simulink library "pwrsysBasic_202301"  (R2018a)
settings: Solver=VariableStepAuto  StartTime=0.0  StopTime=10.0  RelTol=1e-3
values from neighbouring files (symbols this model uses):
  Iap = 1    [SequenceSeparation_script.m]
  Sn = 1.5    [SequenceSeparation_script.m]
  Ts = 1e-6    (= 1e-06)    [SequenceSeparation_script.m]
undefined symbols (not defined in the file or in its folder): DiscIntNeverNeededParam, fn, Kp, tctrl, Uanp
libraries: pwrsysBasic x15, powerlib_meascontrol x12, pwrsysTransf x8, simulink x3
(part 2 of 2)

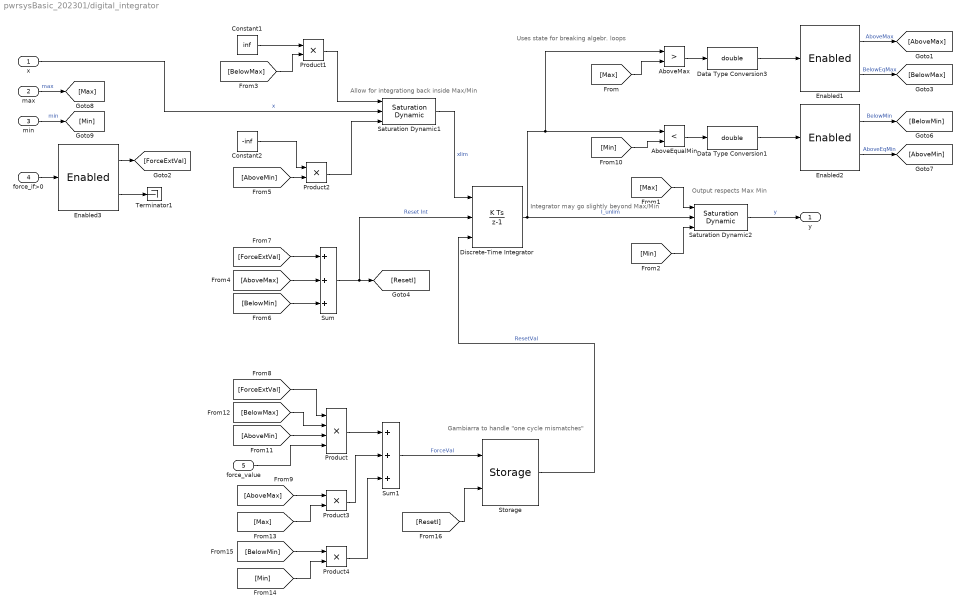
== system pwrsysBasic_202301/digital_integrator ==
  note: Gambiarra to handle "one cycle mismatches"
  note: Integrator may go slightly beyond Max/Min
  note: Output respects Max Min
  note: Uses state for breaking algebr. loops
  note: Allow for integrationg back inside Max/Min
  x : Inport
  max : Inport  Port=2
  min : Inport  Port=3
  force_if>0 : Inport  Port=4
  force_value : Inport  Port=5
  AboveEqualMin : RelationalOperator  Operator=<  OutDataTypeStr=boolean  RndMeth=Nearest
  AboveMax : RelationalOperator  Operator=>  OutDataTypeStr=boolean  RndMeth=Nearest
  Constant1 : Constant  Value=inf
  Constant2 : Constant  Value=-inf
  Data Type Conversion1 : DataTypeConversion  OutDataTypeStr=double
  Data Type Conversion3 : DataTypeConversion  OutDataTypeStr=double
  Discrete-Time Integrator : DiscreteIntegrator  ExternalReset=level  InitialConditionSource=external  SampleTime=Ts  IgnoreLimit=on  ICPrevOutput=DiscIntNeverNeededParam  ICPrevScaledInput=DiscIntNeverNeededParam
  Enabled1 : pwrsysBasic/Enabled
      settings: SourceProductName=NTNU Power Systems
  Enabled2 : pwrsysBasic/Enabled
      settings: SourceProductName=NTNU Power Systems
  Enabled3 : pwrsysBasic/Enabled
      settings: SourceProductName=NTNU Power Systems
  Product : Product  Inputs=4
  Product{1..4} (4 alike) : Product
  Saturation Dynamic1 : simulink/Discontinuities/Saturation Dynamic  OutMin=[]  OutMax=[]  OutDataTypeStr=Inherit: Same as second input  OutDataType=fixdt(1, 16)  OutScaling=2^-10  DoSatur=off
  Saturation Dynamic2 : simulink/Discontinuities/Saturation Dynamic  OutMin=[]  OutMax=[]  OutDataTypeStr=Inherit: Same as second input  OutDataType=fixdt(1, 16)  OutScaling=2^-10  DoSatur=off
  Storage : pwrsysBasic/Storage
      settings: SourceProductName=NTNU Power Systems
  Sum : Sum  Inputs=+++
  Sum1 : Sum  Inputs=+++
  Terminator1 : Terminator
  y : Outport
  wires:
  x/1 -> Saturation Dynamic1/2  "x"
  Saturation Dynamic2/1 -> y/1  "y"
  max/1 -> [Max]  "max"
  min/1 -> [Min]  "min"
  force_value/1 -> Product/4
  Saturation Dynamic1/1 -> Discrete-Time Integrator/1  "xlim"
  [BelowMax] -> Product1/2
  Constant1/1 -> Product1/1
  Product1/1 -> Saturation Dynamic1/1
  [AboveMin] -> Product2/2
  Constant2/1 -> Product2/1
  Product2/1 -> Saturation Dynamic1/3
  Enabled1/1 -> [AboveMax]  "AboveMax"
  Enabled1/2 -> [BelowMax]  "BelowEqMax"
  Enabled2/2 -> [AboveMin]  "AboveEqMin"
  Enabled2/1 -> [BelowMin]  "BelowMin"
  [AboveMax] -> Sum/2
  [BelowMin] -> Sum/3
  force_if>0/1 -> Enabled3/1
  Enabled3/2 -> Terminator1/1
  [ForceExtVal] -> Product/1
  [AboveMax] -> Product3/1
  [Min] -> AboveEqualMin/2
  [AboveMin] -> Product/3
  [BelowMax] -> Product/2
  Product/1 -> Sum1/1
  [Max] -> Product3/2
  [BelowMin] -> Product4/1
  [Min] -> Product4/2
  Product4/1 -> Sum1/3
  Product3/1 -> Sum1/2
  Sum1/1 -> Storage/1  "ForceVal"
  Enabled3/1 -> [ForceExtVal]
  [Max] -> AboveMax/2
  Discrete-Time Integrator/1 -> Saturation Dynamic2/2, AboveEqualMin/1, AboveMax/1  "I_unlim"
  [Max] -> Saturation Dynamic2/1
  [Min] -> Saturation Dynamic2/3
  AboveMax/1 -> Data Type Conversion3/1
  AboveEqualMin/1 -> Data Type Conversion1/1
  Data Type Conversion3/1 -> Enabled1/1
  Data Type Conversion1/1 -> Enabled2/1
  [ForceExtVal] -> Sum/1
  Sum/1 -> Discrete-Time Integrator/2, [ResetI]  "Reset Int"
  [ResetI] -> Storage/2
  Storage/1 -> Discrete-Time Integrator/3  "ResetVal"

== system pwrsysBasic_202301/digital_ramp_gen ==
  up_if>0 : Inport
  down_if>0 : Inport  Port=2
  rate_pu/s : Inport  Port=3
  max : Inport  Port=4
  min : Inport  Port=5
  force_if=1 : Inport  Port=6
  force_value : Inport  Port=7
  Constant : Constant  Value=Ts
  MATLAB Function : MATLAB Function  TreatAsAtomicUnit=on  SystemSampleTime=Ts
      settings: RTWSystemCode=Inline
  y : Outport
  wires:
  up_if>0/1 -> MATLAB Function/1(up)
  MATLAB Function/1(y) -> y/1
  max/1 -> MATLAB Function/4(max)
  min/1 -> MATLAB Function/5(min)
  force_if=1/1 -> MATLAB Function/6(force)
  force_value/1 -> MATLAB Function/7(forceval)
  Constant/1 -> MATLAB Function/8(Ts)
  down_if>0/1 -> MATLAB Function/2(down)
  rate_pu/s/1 -> MATLAB Function/3(rate)

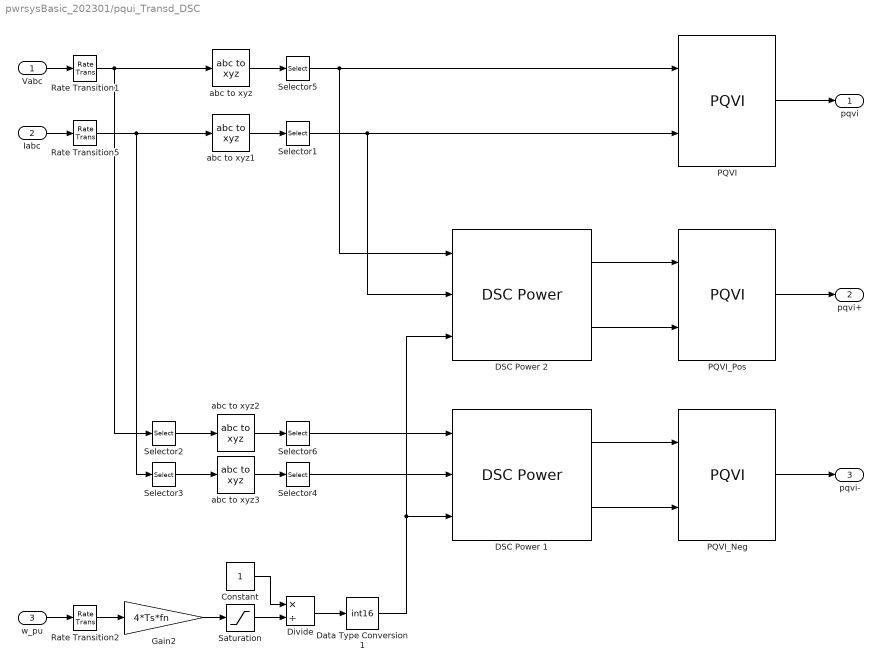
== system pwrsysBasic_202301/pqui_Transd_DSC ==
  Vabc : Inport
  Iabc : Inport  Port=2
  w_pu : Inport  Port=3
  Constant : Constant
  DSC Power 1 : pwrsysBasic/DSC Power 
      settings: SourceProductName=NTNU Power Systems
  DSC Power 2 : pwrsysBasic/DSC Power 
      settings: SourceProductName=NTNU Power Systems
  Data Type Conversion1 : DataTypeConversion  OutDataTypeStr=int16  RndMeth=Round  SaturateOnIntegerOverflow=on
  Divide : Product  Inputs=*/
  Gain2 : Gain  Gain=4*Ts*fn
  PQVI : pwrsysBasic/PQVI  Sn=Sn  Uanp=Uanp  Iap=Iap
      settings: SourceProductName=NTNU Power Systems
  PQVI_Neg : pwrsysBasic/PQVI  Sn=Sn  Uanp=Uanp  Iap=Iap
      settings: SourceProductName=NTNU Power Systems
  PQVI_Pos : pwrsysBasic/PQVI  Sn=Sn  Uanp=Uanp  Iap=Iap
      settings: SourceProductName=NTNU Power Systems
  Rate Transition1 : RateTransition  OutPortSampleTime=Ts
  Rate Transition2 : RateTransition  InitialCondition=1  OutPortSampleTime=Ts
  Rate Transition5 : RateTransition  OutPortSampleTime=Ts
  Saturation : Saturate  UpperLimit=inf  LowerLimit=0.000001
  Selector{1,4..6} (4 alike) : Selector  InputPortWidth=3  IndexOptions=Index vector (dialog)  Indices=[1 2]  OutputSizes=1
  Selector2 : Selector  InputPortWidth=3  IndexOptions=Index vector (dialog)  Indices=[1 3 2]  OutputSizes=1
  Selector3 : Selector  InputPortWidth=3  IndexOptions=Index vector (dialog)  Indices=[1 3 2]  OutputSizes=1
  abc to xyz{,1..3} (4 alike) : pwrsysTransf/abc to xyz  typeTransf=Amplitude-invariant
      settings: SourceProductName=NTNU Power Systems
  pqvi : Outport
  pqvi+ : Outport  Port=2
  pqvi- : Outport  Port=3
  wires:
  abc to xyz1/1 -> Selector1/1
  Vabc/1 -> Rate Transition1/1
  Iabc/1 -> Rate Transition5/1
  Rate Transition1/1 -> abc to xyz/1, Selector2/1
  Rate Transition5/1 -> abc to xyz1/1, Selector3/1
  Selector5/1 -> DSC Power 2/1, PQVI/1
  Selector1/1 -> DSC Power 2/2, PQVI/2
  PQVI/1 -> pqvi/1
  Data Type Conversion1/1 -> DSC Power 1/3, DSC Power 2/3
  DSC Power 2/1 -> PQVI_Pos/1
  DSC Power 2/2 -> PQVI_Pos/2
  PQVI_Pos/1 -> pqvi+/1
  abc to xyz2/1 -> Selector6/1
  abc to xyz3/1 -> Selector4/1
  Selector2/1 -> abc to xyz2/1
  Selector3/1 -> abc to xyz3/1
  Selector6/1 -> DSC Power 1/1
  Selector4/1 -> DSC Power 1/2
  PQVI_Neg/1 -> pqvi-/1
  DSC Power 1/2 -> PQVI_Neg/2
  DSC Power 1/1 -> PQVI_Neg/1
  Saturation/1 -> Divide/2
  Constant/1 -> Divide/1
  Rate Transition2/1 -> Gain2/1
  w_pu/1 -> Rate Transition2/1
  Gain2/1 -> Saturation/1
  Divide/1 -> Data Type Conversion1/1
  abc to xyz/1 -> Selector5/1

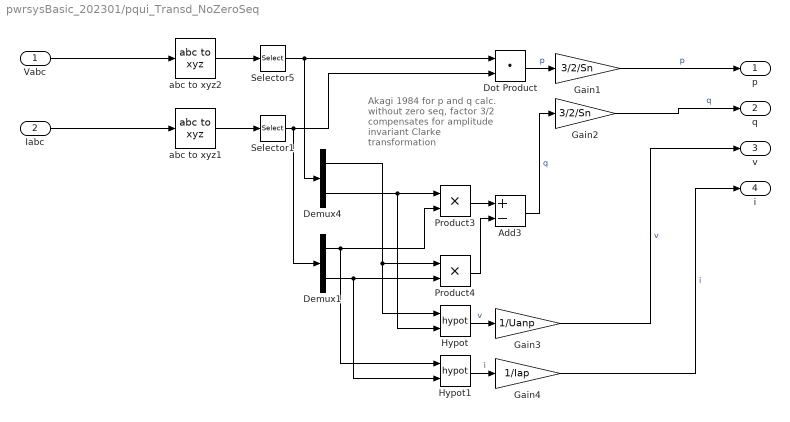
== system pwrsysBasic_202301/pqui_Transd_NoZeroSeq ==
  note: Akagi 1984 for p and q
      | calc. without zero seq,
      | factor 3/2 compensates for
      | amplitude invariant
      | Clarke transformation
  Vabc : Inport
  Iabc : Inport  Port=2
  Add3 : Sum  Inputs=+-
  Demux1 : Demux  Outputs=2
  Demux4 : Demux  Outputs=2
  Dot Product : DotProduct  InputSameDT=on  OutDataTypeStr=Inherit: Inherit via internal rule
  Gain1 : Gain  Gain=3/2/Sn
  Gain2 : Gain  Gain=3/2/Sn
  Gain3 : Gain  Gain=1/Uanp
  Gain4 : Gain  Gain=1/Iap
  Hypot : Math  Operator=hypot  RndMeth=Zero  SaturateOnIntegerOverflow=on
  Hypot1 : Math  Operator=hypot  RndMeth=Zero  SaturateOnIntegerOverflow=on
  Product3 : Product
  Product4 : Product
  Selector1 : Selector  InputPortWidth=3  IndexOptions=Index vector (dialog)  Indices=[1 2]  OutputSizes=1
  Selector5 : Selector  InputPortWidth=3  IndexOptions=Index vector (dialog)  Indices=[1 2]  OutputSizes=1
  abc to xyz1 : pwrsysTransf/abc to xyz  typeTransf=Amplitude-invariant
      settings: SourceProductName=NTNU Power Systems
  abc to xyz2 : pwrsysTransf/abc to xyz  typeTransf=Amplitude-invariant
      settings: SourceProductName=NTNU Power Systems
  p : Outport
  q : Outport  Port=2
  v : Outport  Port=3
  i : Outport  Port=4
  wires:
  abc to xyz1/1 -> Selector1/1
  Gain3/1 -> v/1  "v"
  Demux1/2 -> Hypot1/2, Product4/2
  Hypot1/1 -> Gain4/1  "i"
  Selector1/1 -> Demux1/1, Dot Product/2
  Selector5/1 -> Demux4/1, Dot Product/1
  Demux4/1 -> Hypot/1, Product4/1
  Hypot/1 -> Gain3/1  "v"
  Dot Product/1 -> Gain1/1  "p"
  Demux1/1 -> Hypot1/1, Product3/2
  Add3/1 -> Gain2/1  "q"
  Product4/1 -> Add3/2
  Demux4/2 -> Hypot/2, Product3/1
  Vabc/1 -> abc to xyz2/1
  abc to xyz2/1 -> Selector5/1
  Iabc/1 -> abc to xyz1/1
  Product3/1 -> Add3/1
  Gain1/1 -> p/1  "p"
  Gain4/1 -> i/1  "i"
  Gain2/1 -> q/1  "q"

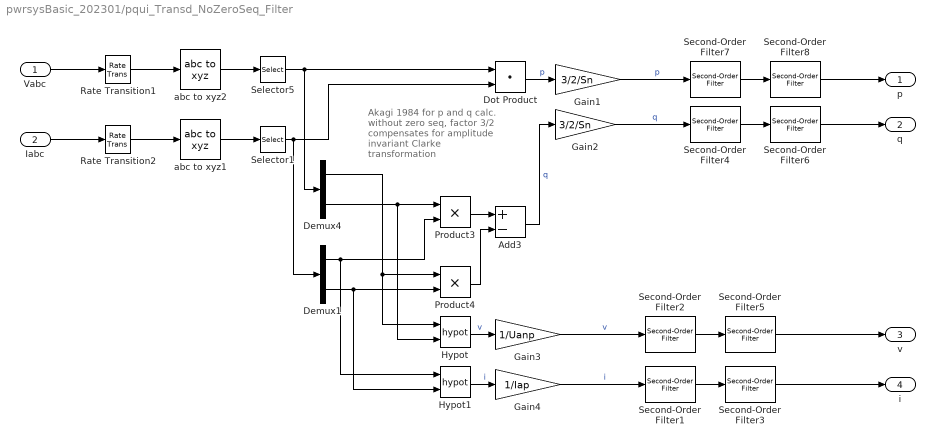
== system pwrsysBasic_202301/pqui_Transd_NoZeroSeq_Filter ==
  note: Akagi 1984 for p and q
      | calc. without zero seq,
      | factor 3/2 compensates for
      | amplitude invariant
      | Clarke transformation
  Vabc : Inport
  Iabc : Inport  Port=2
  Add3 : Sum  Inputs=+-
  Demux1 : Demux  Outputs=2
  Demux4 : Demux  Outputs=2
  Dot Product : DotProduct  InputSameDT=on  OutDataTypeStr=Inherit: Inherit via internal rule
  Gain1 : Gain  Gain=3/2/Sn
  Gain2 : Gain  Gain=3/2/Sn
  Gain3 : Gain  Gain=1/Uanp
  Gain4 : Gain  Gain=1/Iap
  Hypot : Math  Operator=hypot  RndMeth=Zero  SaturateOnIntegerOverflow=on
  Hypot1 : Math  Operator=hypot  RndMeth=Zero  SaturateOnIntegerOverflow=on
  Product3 : Product
  Product4 : Product
  Rate Transition1 : RateTransition  OutPortSampleTime=Ts
  Rate Transition2 : RateTransition  OutPortSampleTime=Ts
  Second-Order Filter1 : powerlib_meascontrol/Filters/Second-Order Filter  FilterType=Lowpass  Fo=fcutoutvi  Zeta=zeta  Ts=Ts  Initialize=off  Vac_Init="[0,  0,  60]"  Vdc_Init=0  PlotResponse=off  FreqRange=[0, 1000, 0.1]
      settings: SourceProductName=Simscape Power Systems  SourceProductBaseCode=PS
  Second-Order Filter2 : powerlib_meascontrol/Filters/Second-Order Filter  FilterType=Lowpass  Fo=fcutoutvi  Zeta=zeta  Ts=Ts  Initialize=off  Vac_Init="[0,  0,  60]"  Vdc_Init=0  PlotResponse=off  FreqRange=[0, 1000, 0.1]
      settings: SourceProductName=Simscape Power Systems  SourceProductBaseCode=PS
  Second-Order Filter{3,5..6,8} (4 alike) : powerlib_meascontrol/Filters/Second-Order Filter  FilterType=Bandstop (Notch)  Fo=fn  Zeta=zeta  Ts=Ts  Initialize=off  Vac_Init="[0,  0,  60]"  Vdc_Init=0  PlotResponse=off  FreqRange=[0, 1000, 0.1]
      settings: SourceProductName=Simscape Power Systems  SourceProductBaseCode=PS
  Second-Order Filter4 : powerlib_meascontrol/Filters/Second-Order Filter  FilterType=Lowpass  Fo=fcutoutpq  Zeta=zeta  Ts=Ts  Initialize=off  Vac_Init="[0,  0,  60]"  Vdc_Init=0  PlotResponse=off  FreqRange=[0, 1000, 0.1]
      settings: SourceProductName=Simscape Power Systems  SourceProductBaseCode=PS
  Second-Order Filter7 : powerlib_meascontrol/Filters/Second-Order Filter  FilterType=Lowpass  Fo=fcutoutpq  Zeta=zeta  Ts=Ts  Initialize=off  Vac_Init="[0,  0,  60]"  Vdc_Init=0  PlotResponse=off  FreqRange=[0, 1000, 0.1]
      settings: SourceProductName=Simscape Power Systems  SourceProductBaseCode=PS
  Selector1 : Selector  InputPortWidth=3  IndexOptions=Index vector (dialog)  Indices=[1 2]  OutputSizes=1
  Selector5 : Selector  InputPortWidth=3  IndexOptions=Index vector (dialog)  Indices=[1 2]  OutputSizes=1
  abc to xyz1 : pwrsysTransf/abc to xyz  typeTransf=Amplitude-invariant
      settings: SourceProductName=NTNU Power Systems
  abc to xyz2 : pwrsysTransf/abc to xyz  typeTransf=Amplitude-invariant
      settings: SourceProductName=NTNU Power Systems
  p : Outport
  q : Outport  Port=2
  v : Outport  Port=3
  i : Outport  Port=4
  wires:
  abc to xyz1/1 -> Selector1/1
  Gain3/1 -> Second-Order Filter2/1  "v"
  Demux1/2 -> Hypot1/2, Product4/2
  Hypot1/1 -> Gain4/1  "i"
  Selector1/1 -> Demux1/1, Dot Product/2
  Selector5/1 -> Demux4/1, Dot Product/1
  Demux4/1 -> Hypot/1, Product4/1
  Hypot/1 -> Gain3/1  "v"
  Iabc/1 -> Rate Transition2/1
  Dot Product/1 -> Gain1/1  "p"
  Demux1/1 -> Hypot1/1, Product3/2
  Add3/1 -> Gain2/1  "q"
  Vabc/1 -> Rate Transition1/1
  Product4/1 -> Add3/2
  Demux4/2 -> Hypot/2, Product3/1
  Rate Transition1/1 -> abc to xyz2/1
  abc to xyz2/1 -> Selector5/1
  Rate Transition2/1 -> abc to xyz1/1
  Product3/1 -> Add3/1
  Gain1/1 -> Second-Order Filter7/1  "p"
  Gain4/1 -> Second-Order Filter1/1  "i"
  Gain2/1 -> Second-Order Filter4/1  "q"
  Second-Order Filter2/1 -> Second-Order Filter5/1
  Second-Order Filter5/1 -> v/1
  Second-Order Filter1/1 -> Second-Order Filter3/1
  Second-Order Filter3/1 -> i/1
  Second-Order Filter4/1 -> Second-Order Filter6/1
  Second-Order Filter6/1 -> q/1
  Second-Order Filter8/1 -> p/1
  Second-Order Filter7/1 -> Second-Order Filter8/1

== system pwrsysBasic_202301/var_delay_floor_ceiling ==
  x(k) : Inport
  n : Inport  Port=2
  S-Function : S-Function  FunctionName=variable_delay_floor_ceil  Parameters=200  SFunctionDeploymentMode=off  EnableBusSupport=off
  x(k-nf) : Outport
  x(k-nc) : Outport  Port=2
  wires:
  n/1 -> S-Function/2
  x(k)/1 -> S-Function/1
  S-Function/1 -> x(k-nf)/1
  S-Function/2 -> x(k-nc)/1

== matlab function pwrsysBasic_202301/digital_ramp_gen/MATLAB Function ==
  data: up input; down input; rate input; y output; max input; min input; force input; forceval input; Ts input
%%%%%%%%%%%%%%%%%%%%%%%%%%%%%%%%%%%%%%%%%%%%%%%%%%%%%%%%%%%%%%%%%%%%%%%%%%
% Digital integrator
%%%%%%%%%%%%%%%%%%%%%%%%%%%%%%%%%%%%%%%%%%%%%%%%%%%%%%%%%%%%%%%%%%%%%%%%%%\
% Forward Euler method: as in matlab help
%   y(n) = y(n-1) + Ts(n-1)*x(n-1)
%   uset it to avoid algebraic loops

% All inputs are stored in states, so there is no direct feedthrough
% GAMBIARRA for avoiding algebraic loops
% see: https://www.mathworks.com/help/simulink/ug/integration-considerations-for-matlab-function-blocks.html

% Inputs
%   up: ramps up
%   down: ramps down (if both up and down, than stops)
%   max: max value for ramp
%   min: min value for ramp
%   force: if=1 sets integrator to forceval
%   forceval: see line above (max and min are respected
%   Ts: sampling time
% Output
%   y: output of the ramp

%%%%%%%%%%%%%%%%%%%%%%%%%%%%%%%%%%%%%%%%%%%%%%%%%%%%%%%%%%%%%%%%%%%%%%%%%%\
% Prog/rev history
%   Mota - 2021-05-21: first release

function y = DigRamp(up, down, rate, max, min, force, forceval, Ts)

% The value of the integrator
persistent i
persistent old_up
persistent old_down
persistent old_rate
persistent old_max
persistent old_min
persistent old_force
persistent old_forceval
persistent old_Ts

% Only at first cycle - outputs zero
if isempty(i)
    y = 0;
    i = 0;
    old_up = 0;
    old_down = 0;
    old_rate = 0;
    old_max = 0;
    old_min = 0;
    old_force = 0;
    old_forceval = 0;
    old_Ts = 0;
    % On the second cycle, output will still be zero, due to choices above
    return;
end

% auxiliary value
aux = 0;

% Bypassing the integrator with a value (can be used for followup)
if old_force == 1
    aux = old_forceval;
else
    %if not bypass, then calculate the next value of the integrator
    aux = i + old_Ts*old_rate*old_up + old_Ts*old_rate*old_down ;
end

%Limiting the integrator
if aux > old_max
    % max value has priority, i.e.,
    % if "max" is below "min" due to engineer error
    % the integrator will stop at "max"
    aux = old_max;
elseif aux < old_min
    % if integrator would cross the min, it will be stopped at min
    aux = old_min;
end

% output of the integrator
y = aux;

%update states
i = aux;
old_rate = rate;
%ramps up if up > 0
if up > 0
    old_up = 1;
else
    old_up = 0;
end
%ramps down if down > 0
if down > 0 
    old_down = -1;
else
    old_down = 0;
end
old_max = max;
old_min = min;
old_force = force;
old_forceval = forceval;
old_Ts = Ts;
